simulink model "Racecar_Pcontroller"  (R2022b)
settings: Solver=VariableStepAuto  StartTime=0.0  StopTime=60  RelTol=1e-3
values from neighbouring files (symbols this model uses):
  x1_0 = 0    [Racecar_Init.m]
  x1_dot_0 = 0    [Racecar_Init.m]
  x2_0 = 0    [Racecar_Init.m]
  x2_dot_0 = 0    [Racecar_Init.m]
settings Model: Creator=logan  LastModifiedBy=logan

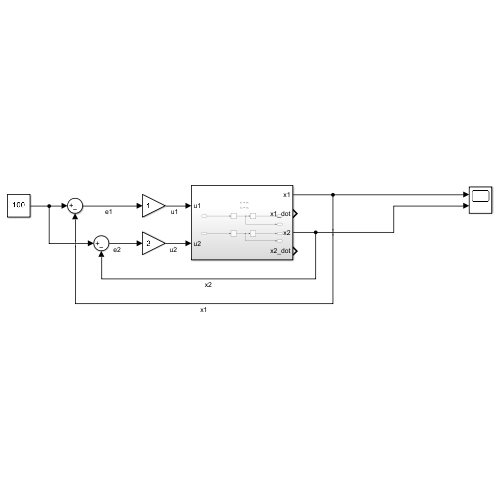
[thumbnail: Simulink's stored preview of the top-level diagram]
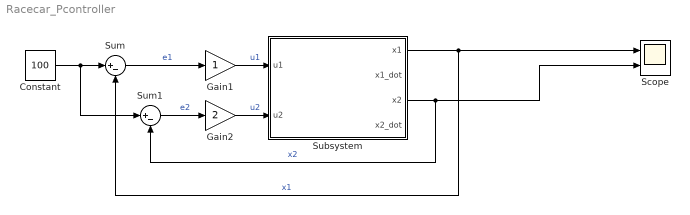
== system Racecar_Pcontroller ==
  Constant : Constant  Value=100
  Gain1 : Gain
  Gain2 : Gain  Gain=2
  Scope : Scope  NumInputPorts=2
  Subsystem : Subsystem
  Sum : Sum  Inputs=|+-
  Sum1 : Sum  Inputs=|+-
  wires:
  Subsystem/1(x1) -> Sum/2, Scope/1  "x1"
  Subsystem/3(x2) -> Sum1/2, Scope/2  "x2"
  Constant/1 -> Sum1/1, Sum/1
  Sum/1 -> Gain1/1  "e1"
  Gain1/1 -> Subsystem/1(u1)  "u1"
  Sum1/1 -> Gain2/1  "e2"
  Gain2/1 -> Subsystem/2(u2)  "u2"

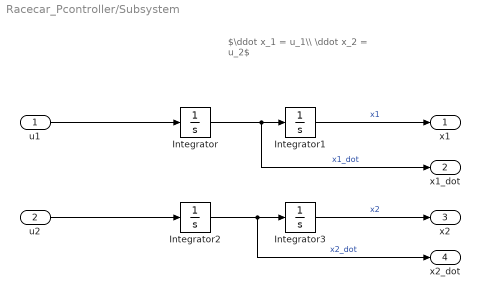
== system Racecar_Pcontroller/Subsystem ==
  note: $\ddot x_1 = u_1\\ \ddot x_2 = u_2$
  u1 : Inport
  u2 : Inport  Port=2
  Integrator : Integrator  InitialCondition=x1_dot_0
  Integrator1 : Integrator  InitialCondition=x1_0
  Integrator2 : Integrator  InitialCondition=x2_dot_0
  Integrator3 : Integrator  InitialCondition=x2_0
  x1 : Outport
  x1_dot : Outport  Port=2
  x2 : Outport  Port=3
  x2_dot : Outport  Port=4
  wires:
  u2/1 -> Integrator2/1
  Integrator2/1 -> x2_dot/1, Integrator3/1  "x2_dot"
  Integrator3/1 -> x2/1  "x2"
  Integrator/1 -> x1_dot/1, Integrator1/1  "x1_dot"
  Integrator1/1 -> x1/1  "x1"
  u1/1 -> Integrator/1
